simulink model "crank_resolved_sidecar"  (R2026a)
settings: Solver=ode3  StopTime=0.9340463713  FixedStep=2e-5
values from neighbouring files (symbols this model uses):
  Eng = struct()    [AeroDieselEngineParameters.m]
libraries: fl_lib x6, nesl_utility x5
settings Model: Creator=asus  LastModifiedBy=asus

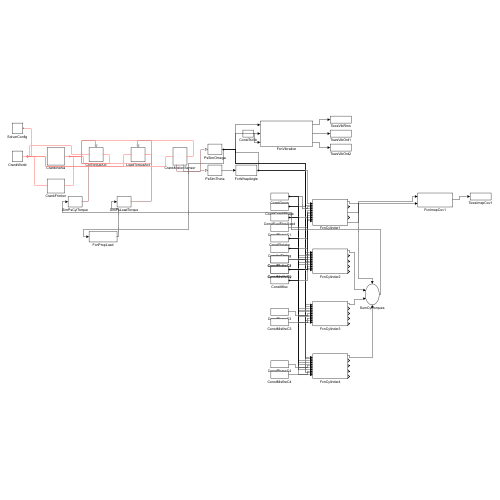
[thumbnail: Simulink's stored preview of the top-level diagram]
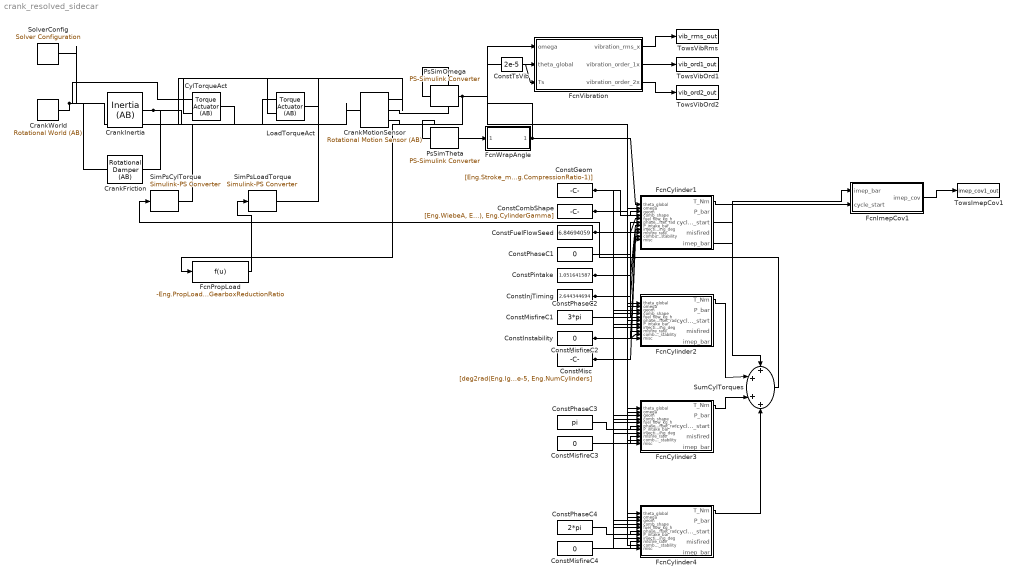
== system crank_resolved_sidecar ==
  ConstCombShape : Constant  Value=[Eng.WiebeA, Eng.WiebeM, deg2rad(Eng.CombustionDuration_deg), Eng.CylinderGamma]
  ConstFuelFlowSeed : Constant  Value=6.84694059
  ConstGeom : Constant  Value=[Eng.Stroke_mm/2000, Eng.ConrodLength_mm/1000, pi/4*(Eng.Bore_mm/1000)^2, (Eng.Displacement_L/1000)/Eng.NumCylinders, ((Eng.Displacement_L/1000)/Eng.NumCylinders)/(Eng.CompressionRatio-1)]
  ConstInjTiming : Constant  Value=2.644344694
  ConstInstability : Constant  Value=0
  ConstMisc : Constant  Value=[deg2rad(Eng.IgnitionDelay_deg), Eng.FuelLHV_MJ_per_kg*1e6, Eng.CombustionEfficiency, Eng.CoolantHeatFraction, 1.0, 2e-5, Eng.NumCylinders]
  ConstMisfireC{1..4} (4 alike) : Constant  Value=0
  ConstPhaseC1 : Constant  Value=0
  ConstPhaseC2 : Constant  Value=3*pi
  ConstPhaseC3 : Constant  Value=pi
  ConstPhaseC4 : Constant  Value=2*pi
  ConstPintake : Constant  Value=1.051641587
  ConstTsVib : Constant  Value=2e-5
  CrankFriction : fl_lib/Rotational/Elements/Rotational Damper (AB)  damping=Eng.FrictionCoeff_Nm_per_rpm*60/(2*pi) N*m*s/rad  t_specify=off  t_priority=None  t=0 N*m  t_nominal_specify=off  t_nominal_value=1  t_nominal_unit=N*m  w_rel_specify=off  w_rel_priority=None  w_rel=0 rad/s  w_rel_nominal_specify=off  w_rel_nominal_value=1  w_rel_nominal_unit=rad/s  theta_rel_specify=off  theta_rel_priority=None  theta_rel=0 rad  theta_rel_nominal_specify=off  theta_rel_nominal_value=1  theta_rel_nominal_unit=rad
  CrankInertia : fl_lib/Rotational/Elements/Inertia (AB)  inertia=Eng.CrankInertia_kgm2 kg*m^2  visible_ports=foundation.enum.RotationalPorts.F  w_specify=on  w_priority=High  w=201.8053546 rad/s  w_nominal_specify=off  w_nominal_value=1  w_nominal_unit=rad/s  t_specify=off  t_priority=None  t=0 N*m  t_nominal_specify=off  t_nominal_value=1  t_nominal_unit=N*m
  CrankMotionSensor : fl_lib/Rotational/Sensors/Rotational Motion Sensor (AB)  reference=foundation.enum.MeasurementReference.difference  acceleration_port=false  velocity_port=true  angle_port=true  wrap_angle=false  wrap_value=0 rad
  CrankWorld : fl_lib/Rotational/Elements/Rotational World (AB)
  CylTorqueAct : fl_lib/Rotational/Sources/Torque Actuator (AB)  theta_rel_specify=off  theta_rel_priority=None  theta_rel=0 rad  theta_rel_nominal_specify=off  theta_rel_nominal_value=1  theta_rel_nominal_unit=rad  t_specify=off  t_priority=None  t=0 N*m  t_nominal_specify=off  t_nominal_value=1  t_nominal_unit=N*m  w_rel_specify=off  w_rel_priority=None  w_rel=0 rad/s  w_rel_nominal_specify=off  w_rel_nominal_value=1  w_rel_nominal_unit=rad/s
  FcnCylinder1 : MATLAB Function  TreatAsAtomicUnit=on  SystemSampleTime=2e-5
  FcnCylinder2 : MATLAB Function  TreatAsAtomicUnit=on  SystemSampleTime=2e-5
  FcnCylinder3 : MATLAB Function  TreatAsAtomicUnit=on  SystemSampleTime=2e-5
  FcnCylinder4 : MATLAB Function  TreatAsAtomicUnit=on  SystemSampleTime=2e-5
  FcnImepCov1 : MATLAB Function  TreatAsAtomicUnit=on  SystemSampleTime=2e-5
  FcnPropLoad : Fcn  Expr=-Eng.PropLoadCoeff_Nm_per_prop_rpm2 * (u*60/(2*pi)/Eng.GearboxReductionRatio)^2 / Eng.GearboxReductionRatio
  FcnVibration : MATLAB Function  TreatAsAtomicUnit=on  SystemSampleTime=2e-5
  FcnWrapAngle : MATLAB Function  TreatAsAtomicUnit=on  SystemSampleTime=2e-5
  LoadTorqueAct : fl_lib/Rotational/Sources/Torque Actuator (AB)  theta_rel_specify=off  theta_rel_priority=None  theta_rel=0 rad  theta_rel_nominal_specify=off  theta_rel_nominal_value=1  theta_rel_nominal_unit=rad  t_specify=off  t_priority=None  t=0 N*m  t_nominal_specify=off  t_nominal_value=1  t_nominal_unit=N*m  w_rel_specify=off  w_rel_priority=None  w_rel=0 rad/s  w_rel_nominal_specify=off  w_rel_nominal_value=1  w_rel_nominal_unit=rad/s
  PsSimOmega : nesl_utility/PS-Simulink Converter  PhysicalDomain=network_engine_domain  SubClassName=ps_output  LeftPortType=input  RightPortType=output  PseudoPeriodic=off  Frequencies=[]  VectorFormat=inherit  Unit=inherit  AffineConversion=off
  PsSimTheta : nesl_utility/PS-Simulink Converter  PhysicalDomain=network_engine_domain  SubClassName=ps_output  LeftPortType=input  RightPortType=output  PseudoPeriodic=off  Frequencies=[]  VectorFormat=inherit  Unit=inherit  AffineConversion=off
  SimPsCylTorque : nesl_utility/Simulink-PS Converter  PhysicalDomain=network_engine_domain  SubClassName=ps_input  LeftPortType=input  RightPortType=output  PseudoPeriodic=off  Frequencies=[]  NoiseDistribution=none  NoiseParameters=[]  Unit=1  AffineConversion=off  FilteringAndDerivatives=provide  SimscapeFilterOrder=1  InputFilterTimeConstant=0.001  UdotUserProvided=0
  SimPsLoadTorque : nesl_utility/Simulink-PS Converter  PhysicalDomain=network_engine_domain  SubClassName=ps_input  LeftPortType=input  RightPortType=output  PseudoPeriodic=off  Frequencies=[]  NoiseDistribution=none  NoiseParameters=[]  Unit=1  AffineConversion=off  FilteringAndDerivatives=provide  SimscapeFilterOrder=1  InputFilterTimeConstant=0.001  UdotUserProvided=0
  SolverConfig : nesl_utility/Solver Configuration  PhysicalDomain=network_engine_domain  SubClassName=solver  LeftPortType=input  RightPortType=generic  Tones=[]  Harmonics=[]  SimulateNoise=off  Profile=off  UseLocalSampling=off  EnableSwitchedLinearOptims=on  FrequencyDomain=off  UseCCode=off  RelTol=0.001  AbsTol=0.001  MinStep=1e-09  ToWorkspace=off  RevertToSquareIcSolve=off  NumHomotopyIterations=100  PhasorMode=off  PhasorModeNumHarmonics=1  ConsistencySolver=NEWTON_XTOL_AFTER_FTOL  CanonicalOrdering=CANONICAL  OptimizeIntermediates=OPTIMIZED  IndexReductionMethod=DerivativeReplacement  DoDC=off  ResidualTolerance=1e-09  ConsistencyTolSource=GLOBAL  ConsistencyAbsTol=0.001  ConsistencyRelTol=0.001  ConsistencyTolFactor=0.001  UseLocalSolver=off  LocalSolverChoice=NE_BACKWARD_EULER_ADVANCER  ResolveIndetEquations=on  FunctionEvalNumThread=1  LocalSolverSampleTime=0.001  DoFixedCost=off  MaxNonlinIter=3  MaxModeIter=2  ComputeImpulses=off  ImpulseIterations=2  LinearAlgebra=auto  LinearAlgebraNumThread=0  EquationFormulation=NE_TIME_EF  DelaysMemoryBudget=1024  AutomaticFiltering=on  FilteringTimeConstant=0.001  PartitionStorageMethod=AS_NEEDED  PartitionMemoryBudget=1024  PartitionMethod=ROBUST  MultibodyUseLocalSolver=off  MultibodyLocalSolverChoice=ODE1  MultibodyLocalSolverSampleTime=0.001
  SumCylTorques : Sum  Inputs=++++
  TowsImepCov1 : ToWorkspace  VariableName=imep_cov1_out  SaveFormat=Timeseries  SampleTime=-1
  TowsVibOrd1 : ToWorkspace  VariableName=vib_ord1_out  SaveFormat=Timeseries  SampleTime=-1
  TowsVibOrd2 : ToWorkspace  VariableName=vib_ord2_out  SaveFormat=Timeseries  SampleTime=-1
  TowsVibRms : ToWorkspace  VariableName=vib_rms_out  SaveFormat=Timeseries  SampleTime=-1
  wires:
  FcnWrapAngle/1(theta_global) -> FcnCylinder1/1(theta_global), FcnCylinder2/1(theta_global), FcnCylinder3/1(theta_global), FcnCylinder4/1(theta_global), FcnVibration/2(theta_global)
  ConstGeom/1 -> FcnCylinder1/3(geom), FcnCylinder2/3(geom), FcnCylinder3/3(geom), FcnCylinder4/3(geom)
  ConstCombShape/1 -> FcnCylinder1/4(comb_shape), FcnCylinder2/4(comb_shape), FcnCylinder3/4(comb_shape), FcnCylinder4/4(comb_shape)
  ConstFuelFlowSeed/1 -> FcnCylinder1/5(fuel_flow_kg_h), FcnCylinder2/5(fuel_flow_kg_h), FcnCylinder3/5(fuel_flow_kg_h), FcnCylinder4/5(fuel_flow_kg_h)
  ConstPhaseC1/1 -> FcnCylinder1/6(phase_offset_rad)
  ConstPintake/1 -> FcnCylinder1/7(P_intake_bar), FcnCylinder2/7(P_intake_bar), FcnCylinder3/7(P_intake_bar), FcnCylinder4/7(P_intake_bar)
  ConstInjTiming/1 -> FcnCylinder1/8(injection_timing_deg), FcnCylinder2/8(injection_timing_deg), FcnCylinder3/8(injection_timing_deg), FcnCylinder4/8(injection_timing_deg)
  ConstMisfireC1/1 -> FcnCylinder1/9(misfire_rate)
  ConstInstability/1 -> FcnCylinder1/10(combustion_stability), FcnCylinder2/10(combustion_stability), FcnCylinder3/10(combustion_stability), FcnCylinder4/10(combustion_stability)
  ConstMisc/1 -> FcnCylinder1/11(misc), FcnCylinder2/11(misc), FcnCylinder3/11(misc), FcnCylinder4/11(misc)
  FcnCylinder1/1(T_Nm) -> SumCylTorques/1
  FcnCylinder1/3(cycle_start) -> FcnImepCov1/2(cycle_start)
  PsSimOmega/1 -> FcnCylinder1/2(omega), FcnCylinder2/2(omega), FcnCylinder3/2(omega), FcnCylinder4/2(omega), FcnPropLoad/1, FcnVibration/1(omega)
  PsSimTheta/1 -> FcnWrapAngle/1(theta_raw)
  ConstPhaseC2/1 -> FcnCylinder2/6(phase_offset_rad)
  ConstMisfireC2/1 -> FcnCylinder2/9(misfire_rate)
  ConstPhaseC3/1 -> FcnCylinder3/6(phase_offset_rad)
  ConstMisfireC3/1 -> FcnCylinder3/9(misfire_rate)
  ConstPhaseC4/1 -> FcnCylinder4/6(phase_offset_rad)
  ConstMisfireC4/1 -> FcnCylinder4/9(misfire_rate)
  FcnCylinder2/1(T_Nm) -> SumCylTorques/2
  FcnCylinder3/1(T_Nm) -> SumCylTorques/3
  FcnCylinder4/1(T_Nm) -> SumCylTorques/4
  SumCylTorques/1 -> SimPsCylTorque/1
  FcnPropLoad/1 -> SimPsLoadTorque/1
  FcnCylinder1/5(imep_bar) -> FcnImepCov1/1(imep_bar)
  FcnImepCov1/1(imep_cov) -> TowsImepCov1/1
  ConstTsVib/1 -> FcnVibration/3(Ts)
  FcnVibration/1(vibration_rms_x) -> TowsVibRms/1
  FcnVibration/2(vibration_order_1x) -> TowsVibOrd1/1
  FcnVibration/3(vibration_order_2x) -> TowsVibOrd2/1
  connections:
  SimPsCylTorque/RConn1 -- CylTorqueAct/LConn2
  SimPsLoadTorque/RConn1 -- LoadTorqueAct/LConn2
  CrankMotionSensor/RConn2 -- PsSimOmega/LConn1
  CrankMotionSensor/RConn3 -- PsSimTheta/LConn1
  CylTorqueAct/RConn1 -- CrankInertia/RConn1 -- CrankFriction/RConn1 -- CrankMotionSensor/RConn1 -- LoadTorqueAct/RConn1
  CylTorqueAct/LConn1 -- SolverConfig/RConn1 -- CrankFriction/LConn1 -- CrankMotionSensor/LConn1 -- CrankWorld/RConn1 -- LoadTorqueAct/LConn1

== matlab function crank_resolved_sidecar/FcnImepCov1 ==
  data: imep_bar input; imep_cov output; cycle_start input
function imep_cov = imepCov(imep_bar, cycle_start)
%#codegen
N = 10;
persistent buf idx count
if isempty(buf)
    buf = zeros(1,N);
    idx = 0;
    count = 0;
end
if cycle_start >= 0.5 && imep_bar ~= 0
    idx = mod(idx, N) + 1;
    buf(idx) = imep_bar;
    count = min(count+1, N);
end
if count >= 2
    valid = buf(1:count);
    m_ = mean(valid);
    if m_ ~= 0
        imep_cov = std(valid)/abs(m_);
    else
        imep_cov = 0;
    end
else
    imep_cov = 0;
end
end

== matlab function crank_resolved_sidecar/FcnVibration ==
  data: omega input; vibration_rms_x output; theta_global input; Ts input; vibration_order_1x output; vibration_order_2x output
function [vibration_rms_x, vibration_order_1x, vibration_order_2x] = vibrationOrderTrack(omega, theta_global, Ts)
%#codegen
persistent last_omega sumsq sumC1 sumS1 sumC2 sumS2 n prev_elapsed theta_start
persistent rms_out ord1_out ord2_out
if isempty(last_omega)
    last_omega = omega;
    sumsq = 0; sumC1 = 0; sumS1 = 0; sumC2 = 0; sumS2 = 0; n = 0;
    theta_start = theta_global;
    prev_elapsed = 0;
    rms_out = 0; ord1_out = 0; ord2_out = 0;
end
vib = (omega - last_omega)/Ts;
last_omega = omega;
theta_mech = mod(theta_global, 2*pi);
sumsq = sumsq + vib^2;
sumC1 = sumC1 + vib*cos(theta_mech);
sumS1 = sumS1 + vib*sin(theta_mech);
sumC2 = sumC2 + vib*cos(2*theta_mech);
sumS2 = sumS2 + vib*sin(2*theta_mech);
n = n + 1;
elapsed = mod(theta_global - theta_start, 4*pi);
if elapsed < prev_elapsed && n > 100
    rms_out = sqrt(sumsq/n);
    ord1_out = 2*sqrt(sumC1^2+sumS1^2)/n;
    ord2_out = 2*sqrt(sumC2^2+sumS2^2)/n;
    sumsq = 0; sumC1 = 0; sumS1 = 0; sumC2 = 0; sumS2 = 0; n = 0;
end
prev_elapsed = elapsed;
vibration_rms_x = rms_out;
vibration_order_1x = ord1_out;
vibration_order_2x = ord2_out;
end

== matlab function crank_resolved_sidecar/FcnCylinder1 ==
  data: theta_global input; T_Nm output; omega input; geom input; comb_shape input; fuel_flow_kg_h input; phase_offset_rad input; P_intake_bar input; injection_timing_deg input; misfire_rate input; combustion_stability input; misc input; P_bar output; cycle_start output; misfired output; imep_bar output
function [T_Nm, P_bar, cycle_start, misfired, imep_bar] = cylinderCombustion(theta_global, omega, geom, comb_shape, fuel_flow_kg_h, phase_offset_rad, P_intake_bar, injection_timing_deg, misfire_rate, combustion_stability, misc)
%#codegen
persistent P prev_in_closed misfired_this_cycle inst_mult_this_cycle work_J_accum imep_bar_out
if isempty(P)
    P = P_intake_bar*1e5;
    prev_in_closed = true;
    misfired_this_cycle = false;
    inst_mult_this_cycle = 1;
    work_J_accum = 0;
    imep_bar_out = 0;
end
a = geom(1); l = geom(2); Area = geom(3); Vd = geom(4);
WiebeA = comb_shape(1); WiebeM = comb_shape(2); dur = comb_shape(3); gamma = comb_shape(4);
ignition_delay = misc(1); LHV = misc(2); CombEff = misc(3); CoolantFrac = misc(4); Patm_bar = misc(5); Ts = misc(6); NumCyl = misc(7);
raw = mod(theta_global - phase_offset_rad, 4*pi);
phi = mod(raw + pi, 4*pi) - pi;
in_closed = (phi <= pi);
cycle_start = 0;
if in_closed && ~prev_in_closed
    if work_J_accum ~= 0
        imep_bar_out = work_J_accum / Vd / 1e5;
    end
    work_J_accum = 0;
    P = P_intake_bar*1e5;
    cycle_start = 1;
    misfired_this_cycle = rand() < misfire_rate;
    inst_mult_this_cycle = 1 + combustion_stability*0.3*randn();
    inst_mult_this_cycle = max(inst_mult_this_cycle, 0);
end
prev_in_closed = in_closed;
misfired = double(misfired_this_cycle);
imep_bar = imep_bar_out;
phi0 = -(deg2rad(injection_timing_deg) - ignition_delay);
if in_closed
    phi_local = phi;
    denom = sqrt(l^2 - a^2*sin(phi_local)^2);
    Vp = geom(5) + Area*(a + l - a*cos(phi_local) - denom);
    dVp = Area*a*sin(phi_local)*(1 + a*cos(phi_local)/denom);
    if phi_local>=phi0 && phi_local<=phi0+dur
        xfrac = max((phi_local-phi0)/dur,0);
        dxdphi_v = WiebeA*(WiebeM+1)/dur * xfrac^WiebeM * exp(-WiebeA*xfrac^(WiebeM+1));
    else
        dxdphi_v = 0;
    end
    fuel_mass_kg = (fuel_flow_kg_h/3600/NumCyl)*(4*pi/omega);
    Qtotal_eff = fuel_mass_kg * LHV * CombEff * (1-CoolantFrac) * inst_mult_this_cycle;
    if misfired_this_cycle
        Qtotal_eff = 0;
    end
    dPdphi = -gamma*P/Vp*dVp + (gamma-1)/Vp*(Qtotal_eff*dxdphi_v);
    dPdt = dPdphi*omega;
    T_Nm = (P - Patm_bar*1e5)*Area*a*(sin(phi_local) + (a*sin(phi_local)*cos(phi_local))/denom);
    work_J_accum = work_J_accum + P*dVp*omega*Ts;
else
    dPdt = 0;
    T_Nm = 0;
end
P = P + Ts*dPdt;
P_bar = P/1e5;
end

== matlab function crank_resolved_sidecar/FcnWrapAngle ==
  data: theta_raw input; theta_global output
function theta_global = wrapAngle(theta_raw)
%#codegen
theta_global = mod(theta_raw, 4*pi);

== matlab function crank_resolved_sidecar/FcnCylinder2 ==
  data: theta_global input; T_Nm output; omega input; geom input; comb_shape input; fuel_flow_kg_h input; phase_offset_rad input; P_intake_bar input; injection_timing_deg input; misfire_rate input; combustion_stability input; misc input; P_bar output; cycle_start output; misfired output; imep_bar output
function [T_Nm, P_bar, cycle_start, misfired, imep_bar] = cylinderCombustion(theta_global, omega, geom, comb_shape, fuel_flow_kg_h, phase_offset_rad, P_intake_bar, injection_timing_deg, misfire_rate, combustion_stability, misc)
%#codegen
persistent P prev_in_closed misfired_this_cycle inst_mult_this_cycle work_J_accum imep_bar_out
if isempty(P)
    P = P_intake_bar*1e5;
    prev_in_closed = true;
    misfired_this_cycle = false;
    inst_mult_this_cycle = 1;
    work_J_accum = 0;
    imep_bar_out = 0;
end
a = geom(1); l = geom(2); Area = geom(3); Vd = geom(4);
WiebeA = comb_shape(1); WiebeM = comb_shape(2); dur = comb_shape(3); gamma = comb_shape(4);
ignition_delay = misc(1); LHV = misc(2); CombEff = misc(3); CoolantFrac = misc(4); Patm_bar = misc(5); Ts = misc(6); NumCyl = misc(7);
raw = mod(theta_global - phase_offset_rad, 4*pi);
phi = mod(raw + pi, 4*pi) - pi;
in_closed = (phi <= pi);
cycle_start = 0;
if in_closed && ~prev_in_closed
    if work_J_accum ~= 0
        imep_bar_out = work_J_accum / Vd / 1e5;
    end
    work_J_accum = 0;
    P = P_intake_bar*1e5;
    cycle_start = 1;
    misfired_this_cycle = rand() < misfire_rate;
    inst_mult_this_cycle = 1 + combustion_stability*0.3*randn();
    inst_mult_this_cycle = max(inst_mult_this_cycle, 0);
end
prev_in_closed = in_closed;
misfired = double(misfired_this_cycle);
imep_bar = imep_bar_out;
phi0 = -(deg2rad(injection_timing_deg) - ignition_delay);
if in_closed
    phi_local = phi;
    denom = sqrt(l^2 - a^2*sin(phi_local)^2);
    Vp = geom(5) + Area*(a + l - a*cos(phi_local) - denom);
    dVp = Area*a*sin(phi_local)*(1 + a*cos(phi_local)/denom);
    if phi_local>=phi0 && phi_local<=phi0+dur
        xfrac = max((phi_local-phi0)/dur,0);
        dxdphi_v = WiebeA*(WiebeM+1)/dur * xfrac^WiebeM * exp(-WiebeA*xfrac^(WiebeM+1));
    else
        dxdphi_v = 0;
    end
    fuel_mass_kg = (fuel_flow_kg_h/3600/NumCyl)*(4*pi/omega);
    Qtotal_eff = fuel_mass_kg * LHV * CombEff * (1-CoolantFrac) * inst_mult_this_cycle;
    if misfired_this_cycle
        Qtotal_eff = 0;
    end
    dPdphi = -gamma*P/Vp*dVp + (gamma-1)/Vp*(Qtotal_eff*dxdphi_v);
    dPdt = dPdphi*omega;
    T_Nm = (P - Patm_bar*1e5)*Area*a*(sin(phi_local) + (a*sin(phi_local)*cos(phi_local))/denom);
    work_J_accum = work_J_accum + P*dVp*omega*Ts;
else
    dPdt = 0;
    T_Nm = 0;
end
P = P + Ts*dPdt;
P_bar = P/1e5;
end

== matlab function crank_resolved_sidecar/FcnCylinder3 ==
  data: theta_global input; T_Nm output; omega input; geom input; comb_shape input; fuel_flow_kg_h input; phase_offset_rad input; P_intake_bar input; injection_timing_deg input; misfire_rate input; combustion_stability input; misc input; P_bar output; cycle_start output; misfired output; imep_bar output
function [T_Nm, P_bar, cycle_start, misfired, imep_bar] = cylinderCombustion(theta_global, omega, geom, comb_shape, fuel_flow_kg_h, phase_offset_rad, P_intake_bar, injection_timing_deg, misfire_rate, combustion_stability, misc)
%#codegen
persistent P prev_in_closed misfired_this_cycle inst_mult_this_cycle work_J_accum imep_bar_out
if isempty(P)
    P = P_intake_bar*1e5;
    prev_in_closed = true;
    misfired_this_cycle = false;
    inst_mult_this_cycle = 1;
    work_J_accum = 0;
    imep_bar_out = 0;
end
a = geom(1); l = geom(2); Area = geom(3); Vd = geom(4);
WiebeA = comb_shape(1); WiebeM = comb_shape(2); dur = comb_shape(3); gamma = comb_shape(4);
ignition_delay = misc(1); LHV = misc(2); CombEff = misc(3); CoolantFrac = misc(4); Patm_bar = misc(5); Ts = misc(6); NumCyl = misc(7);
raw = mod(theta_global - phase_offset_rad, 4*pi);
phi = mod(raw + pi, 4*pi) - pi;
in_closed = (phi <= pi);
cycle_start = 0;
if in_closed && ~prev_in_closed
    if work_J_accum ~= 0
        imep_bar_out = work_J_accum / Vd / 1e5;
    end
    work_J_accum = 0;
    P = P_intake_bar*1e5;
    cycle_start = 1;
    misfired_this_cycle = rand() < misfire_rate;
    inst_mult_this_cycle = 1 + combustion_stability*0.3*randn();
    inst_mult_this_cycle = max(inst_mult_this_cycle, 0);
end
prev_in_closed = in_closed;
misfired = double(misfired_this_cycle);
imep_bar = imep_bar_out;
phi0 = -(deg2rad(injection_timing_deg) - ignition_delay);
if in_closed
    phi_local = phi;
    denom = sqrt(l^2 - a^2*sin(phi_local)^2);
    Vp = geom(5) + Area*(a + l - a*cos(phi_local) - denom);
    dVp = Area*a*sin(phi_local)*(1 + a*cos(phi_local)/denom);
    if phi_local>=phi0 && phi_local<=phi0+dur
        xfrac = max((phi_local-phi0)/dur,0);
        dxdphi_v = WiebeA*(WiebeM+1)/dur * xfrac^WiebeM * exp(-WiebeA*xfrac^(WiebeM+1));
    else
        dxdphi_v = 0;
    end
    fuel_mass_kg = (fuel_flow_kg_h/3600/NumCyl)*(4*pi/omega);
    Qtotal_eff = fuel_mass_kg * LHV * CombEff * (1-CoolantFrac) * inst_mult_this_cycle;
    if misfired_this_cycle
        Qtotal_eff = 0;
    end
    dPdphi = -gamma*P/Vp*dVp + (gamma-1)/Vp*(Qtotal_eff*dxdphi_v);
    dPdt = dPdphi*omega;
    T_Nm = (P - Patm_bar*1e5)*Area*a*(sin(phi_local) + (a*sin(phi_local)*cos(phi_local))/denom);
    work_J_accum = work_J_accum + P*dVp*omega*Ts;
else
    dPdt = 0;
    T_Nm = 0;
end
P = P + Ts*dPdt;
P_bar = P/1e5;
end

== matlab function crank_resolved_sidecar/FcnCylinder4 ==
  data: theta_global input; T_Nm output; omega input; geom input; comb_shape input; fuel_flow_kg_h input; phase_offset_rad input; P_intake_bar input; injection_timing_deg input; misfire_rate input; combustion_stability input; misc input; P_bar output; cycle_start output; misfired output; imep_bar output
function [T_Nm, P_bar, cycle_start, misfired, imep_bar] = cylinderCombustion(theta_global, omega, geom, comb_shape, fuel_flow_kg_h, phase_offset_rad, P_intake_bar, injection_timing_deg, misfire_rate, combustion_stability, misc)
%#codegen
persistent P prev_in_closed misfired_this_cycle inst_mult_this_cycle work_J_accum imep_bar_out
if isempty(P)
    P = P_intake_bar*1e5;
    prev_in_closed = true;
    misfired_this_cycle = false;
    inst_mult_this_cycle = 1;
    work_J_accum = 0;
    imep_bar_out = 0;
end
a = geom(1); l = geom(2); Area = geom(3); Vd = geom(4);
WiebeA = comb_shape(1); WiebeM = comb_shape(2); dur = comb_shape(3); gamma = comb_shape(4);
ignition_delay = misc(1); LHV = misc(2); CombEff = misc(3); CoolantFrac = misc(4); Patm_bar = misc(5); Ts = misc(6); NumCyl = misc(7);
raw = mod(theta_global - phase_offset_rad, 4*pi);
phi = mod(raw + pi, 4*pi) - pi;
in_closed = (phi <= pi);
cycle_start = 0;
if in_closed && ~prev_in_closed
    if work_J_accum ~= 0
        imep_bar_out = work_J_accum / Vd / 1e5;
    end
    work_J_accum = 0;
    P = P_intake_bar*1e5;
    cycle_start = 1;
    misfired_this_cycle = rand() < misfire_rate;
    inst_mult_this_cycle = 1 + combustion_stability*0.3*randn();
    inst_mult_this_cycle = max(inst_mult_this_cycle, 0);
end
prev_in_closed = in_closed;
misfired = double(misfired_this_cycle);
imep_bar = imep_bar_out;
phi0 = -(deg2rad(injection_timing_deg) - ignition_delay);
if in_closed
    phi_local = phi;
    denom = sqrt(l^2 - a^2*sin(phi_local)^2);
    Vp = geom(5) + Area*(a + l - a*cos(phi_local) - denom);
    dVp = Area*a*sin(phi_local)*(1 + a*cos(phi_local)/denom);
    if phi_local>=phi0 && phi_local<=phi0+dur
        xfrac = max((phi_local-phi0)/dur,0);
        dxdphi_v = WiebeA*(WiebeM+1)/dur * xfrac^WiebeM * exp(-WiebeA*xfrac^(WiebeM+1));
    else
        dxdphi_v = 0;
    end
    fuel_mass_kg = (fuel_flow_kg_h/3600/NumCyl)*(4*pi/omega);
    Qtotal_eff = fuel_mass_kg * LHV * CombEff * (1-CoolantFrac) * inst_mult_this_cycle;
    if misfired_this_cycle
        Qtotal_eff = 0;
    end
    dPdphi = -gamma*P/Vp*dVp + (gamma-1)/Vp*(Qtotal_eff*dxdphi_v);
    dPdt = dPdphi*omega;
    T_Nm = (P - Patm_bar*1e5)*Area*a*(sin(phi_local) + (a*sin(phi_local)*cos(phi_local))/denom);
    work_J_accum = work_J_accum + P*dVp*omega*Ts;
else
    dPdt = 0;
    T_Nm = 0;
end
P = P + Ts*dPdt;
P_bar = P/1e5;
end
